simulink library "Min_Run_Time"  (Simulink 8.2)
settings: Solver=ode45  StartTime=0.0  StopTime=10.0  RelTol=1e-3
libraries: simulink x1
settings Model: Creator=lena.frank  LastModifiedBy=drhf

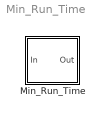
== system Min_Run_Time ==
  Min_Run_Time : Subsystem  mask(Minimum Running Time){tminrun=2, mv=2}
      mask prompts: tminrun "Minimum operation time in s"; mv "Minimum output value"
      mask help: Once started, the output is kept to the maximum of the input value and the mimimum output for at least the minimum running time.
      mask Help: web(fullfile(path_carnot('help'),'Min_Run_Time.html'),'-helpbrowser')
      mask Display:
      | plot(-20,-30,120,100,[10,20,40,60,80,90,90,80,60,40,20,10,10],[40,20,10,10,20,40,60,80,90,90,80,60,40],[55,46],[95,95],[50,50],[90,95],[50,50,24],[88,50,66],[10,13],[50,50],[90,87],[50,50],[50,50],[10,15])
      | disp('\n\nMin On')

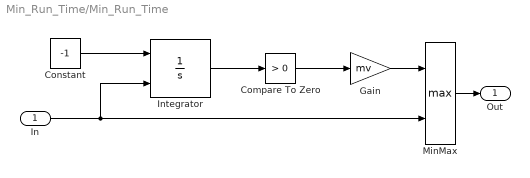
== system Min_Run_Time/Min_Run_Time ==
  In : Inport
  Compare To Zero : simulink/Logic and Bit Operations/Compare To Zero  relop=>  OutDataTypeStr=uint8
  Constant : Constant  Value=-1
  Gain : Gain  Gain=mv
  Integrator : Integrator  ExternalReset=rising  InitialCondition=tminrun  LimitOutput=on  LowerSaturationLimit=0
  MinMax : MinMax  Function=max  Inputs=2
  Out : Outport
  wires:
  Gain/1 -> MinMax/1
  Constant/1 -> Integrator/1
  Integrator/1 -> Compare To Zero/1
  Compare To Zero/1 -> Gain/1
  In/1 -> Integrator/2, MinMax/2
  MinMax/1 -> Out/1
